simulink model "HEV_SeriesParallel"  (R2016b)
settings: Solver=ode15s  StartTime=0.0  StopTime=195  RelTol=1e-4  AbsTol=1e-5  EnableMultiTasking=on
PreLoadFcn:
  | load UrbanCycle1
  | load UrbanCycle2
  | load UrbanCycle3
  | load UrbanCycle4
  | load UrbanCycle5
  | 
  | assignin('base','decimation',1)
  | Pbatt = 21e3;
  | Vbatt =100;
  | Ts = 6e-5;   % time step
  | 
  | Drive_Cycle_Num = 1;
  | warning off Simulink:Commands:LoadMdlParameterizedLink
PostLoadFcn:
  | warning off Simulink:Engine:UsingDefaultMaxStepSize
  | warning off Simulink:blocks:MatchingGotoNotFound
  | warning off Simulink:blocks:MatchingFromNotFound
  | warning off Simulink:blocks:TDelayBufferTooSmall
  | warning off Simulink:SL_SaveWithParameterizedLinks_Warning
  | warning off Simulink:SL_TDelayBufferTooSmall
  | warning off Simulink:SL_OutputNotConnected
  | warning off Simulink:SL_SaveWithDisabledLinks_Warning
  | 
  | warning off Simulink:SL_SetParamLinkChangeWarn
  | 
  | warning('off','Simulink:SL_UINotUpdatedDuringRapidAccelSim');
  | warning off Simulink:Engine:OutputNotConnected
  | warning off Simulink:Engine:UINotUpdatedDuringRapidAccelSim
  | warning off Simulink:Engine:SaveWithParameterizedLinks_Warning
  | warning off Simulink:Engine:SolverMaskedZC
  | set_param('HEV_SeriesParallel','MaskedZcDiagnostic','none');
  | warning off Simulink:Engine:SolverInconsistentInitialConditionsWarnForDAE
  | set_param('HEV_SeriesParallel','IgnoredZcDiagnostic','none');
  | warning off Simulink:Engine:SolverIgnoredZCBracketing
  | set_param('HEV_SeriesParallel','MaxConsecutiveZCsMsg','none');
  | warning off Simulink:Engine:SolverConsecutiveZCNum
  | warning off Simulink:Engine:SolverMinStepSizeWarnForDAE
  | warning off Simulink:Engine:SolverMinStepNonlinearIterWarnForDAE
  | warning off simscape:compiler:sli:init:SolverNotRecommended
  | warning off Simulink:Commands:SetParamLinkChangeWarn
  | warning off xPCTarget:sampleTime:sampleTimeInvariance
  | warning off Simulink:blocks:TDelayFixedBuffer
  | 
  | Setup_HEV_Model_Configurations
  | 
  | % Commands to avoid warning at first run
  | % PS battery function
  | warning off MATLAB:illConditionedMatrix
  | try
  |    set_param(bdroot, 'SimulationCommand', 'update');
  | catch
  | end
  | warning on MATLAB:illConditionedMatrix
InitFcn:
  | Configure_HEV_Simulation
StartFcn:
  | tic;
StopFcn:
  | Elapsed_Sim_Time = toc; disp(['Elapsed time for ' bdroot ' = ' num2str(Elapsed_Sim_Time)])
model workspace (MAT data in the model file):
  guiH = 18054.0001221
undefined symbols (not defined in the file): drive_block, drive_enginemodel, HEV_Param, sigbuilder_block, speed, torque
libraries: fl_lib x18, nesl_utility x11, HEV_Electrical_Lib x3, sdl_lib x2, HEV_Vehicle_Dynamics_Lib x2, simulink x1, slrtlib x1, powerlib x1
(part 2 of 2)

== system HEV_SeriesParallel/Control/Engine Speed Controller/Engine Running/Alternate Logic ==
  RPM Dem : Inport
  Allow time for engine to start : TransportDelay
  No delay for engine stopping : Product  RndMeth=Zero
  Start engine : Fcn  Expr=u(1) > HEV_Param.Control.Engine_Start_RPM
  ICE Enable : Outport
  wires:
  Start engine/1 -> Allow time for engine to start/1, No delay for engine stopping/2
  Allow time for engine to start/1 -> No delay for engine stopping/1
  RPM Dem/1 -> Start engine/1
  No delay for engine stopping/1 -> ICE Enable/1

== stateflow chart HEV_SeriesParallel/Control/Mode Logic ==
  settings: updateMethod=DISCRETE  sampleTime=HEV_Param.Control.Mode_Logic_TS
  state Motion_mode
    state Start_mode
      entry: Gen_Enable=1;
      Mot_Enable=1;
      ICE_Enable=0;
    state Normal_mode
      entry: ICE_Enable=1;
      state Accelerate_mode
        entry: Gen_Enable=0;
        Mot_Enable=1;
      state Cruise_mode
        entry: Mot_Enable=1;
        state charge
          entry:Gen_Enable=1;
        state nocharge
          entry:Gen_Enable=0;
        (default) -> charge
        charge -> nocharge : [charge>99.9]
        nocharge -> charge : [charge<30]
      (default) -> Accelerate_mode
      Cruise_mode -> Accelerate_mode : [(speed <0.998*oldspeed() ...
          | || speed>1.002*oldspeed()) ...
          | && charge>30]
      Accelerate_mode -> Cruise_mode : [(speed >0.998*oldspeed() ...
          |  && speed<1.002* ...
          | oldspeed())|| charge<=30]
    (default) -> Start_mode
    Normal_mode -> Start_mode : [engine_speed<=EngOffRPM]
    Start_mode -> Normal_mode : [engine_speed>EngOnRPM]
  state Brake_mode
    entry: Mot_Enable=1;
    Gen_Enable=0;
    ICE_Enable=0;
  (default) -> Motion_mode
  Motion_mode -> Brake_mode : [brake>=0.05]
  Brake_mode -> Motion_mode : [brake<0.05]
  data: y function_output double; speed input; Mot_Enable output double; Gen_Enable output double; brake input; speed_buffer local double size=21; ICE_Enable output double; charge input; engine_speed input; EngOnRPM constant double =HEV_Param.Control.Engine_Start_RPM; EngOffRPM constant double =HEV_Param.Control.Engine_Stop_RPM
  function y = oldspeed:
    | function y = oldspeed
    | speed_buffer(2:end) = speed_buffer(1:end-1);
    | speed_buffer(1) = speed;
    | y = mean(speed_buffer);
